simulink model "Vehicle_dynamics"  (R2022a)
settings: Solver=VariableStepAuto  StartTime=0.0  StopTime=20  RelTol=1e-3
undefined symbols (not defined in the file or in its folder): deg, driving, rad, s
libraries: drivingscenarioandsensors x2, simulink_extras x2, autolibshared x2, aerolibconvert2 x1, vehdynlibsteering x1
settings Model: Creator=User  LastModifiedBy=User

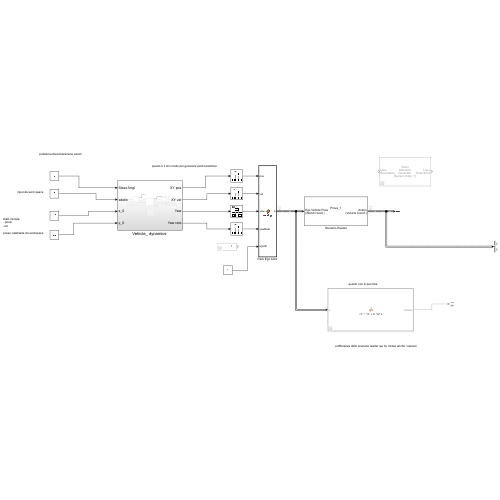
[thumbnail: Simulink's stored preview of the top-level diagram]
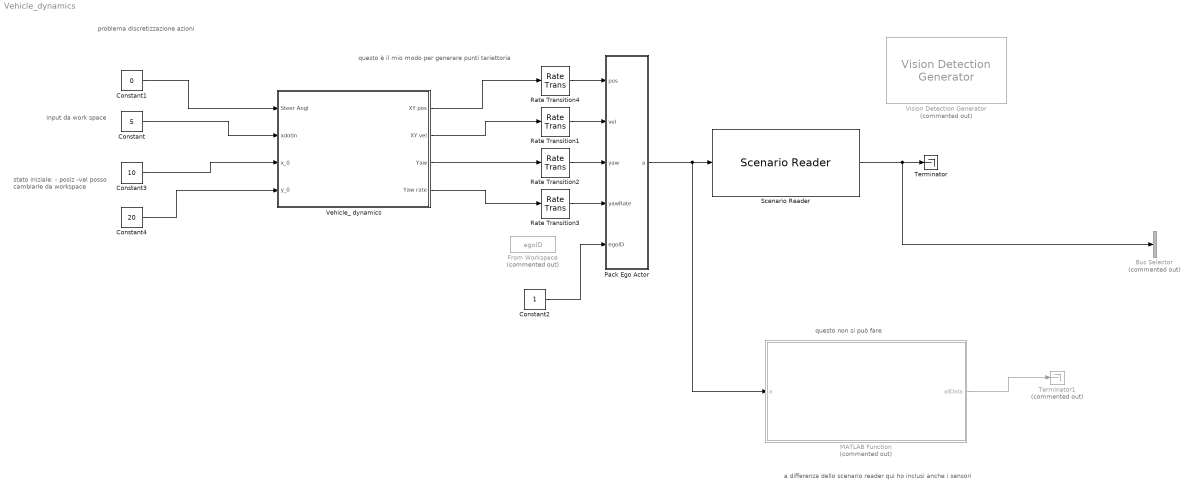
== system Vehicle_dynamics ==
  note: input da work space
  note: questo è il mio modo per generare punti tariettoria
  note: questo non si può fare
  note: a differenza dello scenario reader qui ho inclusi anche i sensori
  note: problema discretizzazione azioni
  note: stato iniziale:
      | - posiz
      | -vel
      |
      | posso cambiarle da workspace
  Bus Selector : BusSelector  Commented=on  OutputSignals=signal1,signal2
  Constant : Constant  Value=5
  Constant1 : Constant  Value=0
  Constant2 : Constant
  Constant3 : Constant  Value=10
  Constant4 : Constant  Value=20
  From Workspace : FromWorkspace  Commented=on  VariableName=egoID
  MATLAB Function : MATLAB Function  Commented=on  TreatAsAtomicUnit=on
  Pack Ego Actor : MATLAB Function  TreatAsAtomicUnit=on
  Rate Transition{1..4} (4 alike) : RateTransition  OutPortSampleTime=Ts
  Scenario Reader : drivingscenarioandsensors/Scenario Reader  ScenarioSource=From file  ScenarioFileName=C:\Users\User\OneDrive\Desktop\Thesis\Codice\Prova_1.mat  ScenarioVariableName=scenario  OutputCoordinateSystem=Vehicle coordinates  EgoVehicleSource=Input port  EgoVehicleActorID=1  OrientVehiclesOnRoad=off  OutputEgoVehiclePose=off  OutputEgoVehicleState=off  SampleTime=0.1  LaneBoundaryOutput=None  LaneBoundaryDistance=0:0.5:9.5  LaneBoundaryLocation=Center of lane markings  BusNameSource=Auto  BusName=BusActors  BusNumActorsSource=Scenario  BusNumActors=100  BusName2Source=Auto  BusName2=BusLaneBoundaries  BusNumLaneBoundariesSource=Scenario  BusNumLaneBoundaries=10  BusName3Source=Auto  BusName3=BusEgoActor  BusName4Source=Auto  BusName4=BusEgoState  ShowCoordinateLabels=on  SimulateUsing=Interpreted execution
  Terminator : Terminator
  Terminator1 : Terminator  Commented=on
  "Vehicle_ dynamics " : Subsystem
  Vision Detection Generator : drivingscenarioandsensors/Vision Detection Generator  Commented=on  SensorIndex=1  DetectorOutput=Lanes only  UpdateInterval=0.1  LaneUpdateInterval=0.1  SensorLocation=[ 1.9, 0 ]  Height=1.1  Yaw=0  Pitch=1  Roll=0  BusNameSource=Auto  BusName=BusObjectDetections  BusName2Source=Auto  BusName2=BusLaneDetections  MaxNumDetectionsSource=Property  MaxNumDetections=50  MaxNumLanesSource=Property  MaxNumLanes=30  DetectionCoordinates=Ego Cartesian  SimulateUsing=Interpreted execution  MaxRange=150  BoundingBoxAccuracy=5  ProcessNoiseIntensity=5  MaxSpeed=100  MaxAllowedOcclusion=0.5  MinObjectImageSize=[ 15, 15 ]  DetectionProbability=0.9  FalsePositivesPerImage=0.1  MinLaneImageSize=[ 20, 3 ]  LaneBoundaryAccuracy=3  HasNoise=on  InitialSeedSource=Repeatable  InitialSeed=0  UsedSeed=driving.internal.SimulinkUtilities.seedManager(gcb)  ActorProfilesSource=From Scenario Reader block  ActorProfilesParameters=driving.internal.ActorProfilesParameters  ActorProfilesExpression=struct( 'ClassID', 0, 'Length', 4.7, 'Width', 1.8, 'Height', 1.4, 'OriginOffset', [ -1.35, 0, 0 ] )  Intrinsics=driving.internal.cameraIntrinsics
  wires:
  Constant1/1 -> "Vehicle_ dynamics "/1(Steer Angl)
  Constant/1 -> "Vehicle_ dynamics "/2(xdotin)
  Rate Transition4/1 -> Pack Ego Actor/1(pos)
  Rate Transition1/1 -> Pack Ego Actor/2(vel)
  Rate Transition2/1 -> Pack Ego Actor/3(yaw)
  Rate Transition3/1 -> Pack Ego Actor/4(yawRate)
  "Vehicle_ dynamics "/1(XY pos) -> Rate Transition4/1
  "Vehicle_ dynamics "/2(XY vel) -> Rate Transition1/1
  "Vehicle_ dynamics "/4(Yaw rate) -> Rate Transition3/1
  Constant2/1 -> Pack Ego Actor/5(egoID)
  "Vehicle_ dynamics "/3(Yaw) -> Rate Transition2/1
  Pack Ego Actor/1(a) -> MATLAB Function/1(a), Scenario Reader/1
  Scenario Reader/1 -> Bus Selector/1, Terminator/1
  Constant3/1 -> "Vehicle_ dynamics "/3(x_0)
  Constant4/1 -> "Vehicle_ dynamics "/4(y_0)
  MATLAB Function/1(allData) -> Terminator1/1

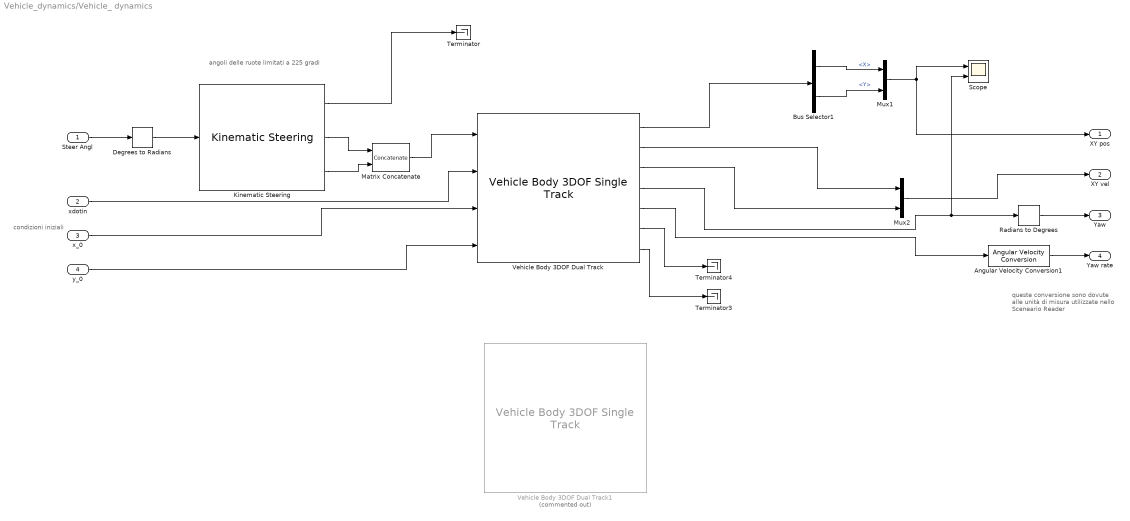
== system Vehicle_dynamics/Vehicle_ dynamics  ==
  note: angoli delle ruote limitati a 225 gradi
  note: condizioni
      | iniziali
  note: queste conversione sono dovute
      | alle unità di misura utilizzate nello
      | Sceneario Reader
  Steer Angl : Inport
  xdotin : Inport  Port=2
  x_0 : Inport  Port=3
  y_0 : Inport  Port=4
  Angular Velocity Conversion1 : aerolibconvert2/Angular Velocity Conversion  IU=rad/s  OU=deg/s
  Bus Selector1 : BusSelector  OutputSignals=InertFrm.Cg.Disp.X,InertFrm.Cg.Disp.Y
  Degrees to Radians : simulink_extras/Transformations/Degrees to Radians
  Kinematic Steering : vehdynlibsteering/Kinematic Steering  StrgType=Ackerman  StrgRatioType=Constant  Loc=Front  NrmlFctr=0.01  TrckWdth=1  WhlBase=1.524  Db=0  StrgRng=1.25*pi  StrgAngBpts="[-6.2832   -5.0265   -3.7699   -2.5133   -1.2566         0    1.2566    2.5133    3.7699    5.0265    6.2832]"  StrgRatioTbl=|  StrgRatio=100  PctAckIn=off  PctAck=100  PctAckTbl=ones(1,11)*100  StrgArmLngth=0.1  RckCsLngth=0.5  TieRodLngth=0.248  D=0.2  PnnRadius=0.00085818  PnnRadiusTbl="[0.0055    0.0055    0.0056    0.0057    0.0058    0.0057    0.0057    0.0057    0.0056    0.0055    0.0055]"  RodLngth=0.1  ParaArmLngth=0.9  aMode=2
      | [13.5000   13.3750   13.2500   13.1250   13.0000   13.0000   13.0000   13.1250   13.2500   13.3750   13.5000
      | ]
  Matrix Concatenate : Concatenate  ConcatenateDimension=2
  Mux1 : Mux  Inputs=2
  Mux2 : Mux  Inputs=2
  Radians to Degrees : simulink_extras/Transformations/Radians to Degrees
  Scope : Scope  NumInputPorts=2
  Terminator : Terminator
  Terminator3 : Terminator
  Terminator4 : Terminator
  Vehicle Body 3DOF Dual Track : autolibshared/Vehicle Body 3DOF Single Track  trackMode=Dual  inputMode=External longitudinal velocity  frontSteerMode=on  rearSteerMode=off  windMode=off  muMode=off  extFMode=off  extMMode=off  htchFMode=off  htchMMode=off  extXo=on  extpsio=off  extxdoto=off  extro=off  extYo=on  extTamb=off  extydoto=off  aMode=2  NF=2  NR=2  m=2000  a=1.4  b=1.6  h=0.35  dh=1  hh=0.2  X_o=0  xdot_o=0  CalphaMode=off  sigmaMode=on  d=0  hl=0  w=[1.4,1.4]  Cy_f=12e3  Cy_r=11e3  sigma_f=.1  sigma_r=.1  alpha_f_brk=[-.1 .1]  Cy_f_data=[-9e3 9e3]  alpha_r_brk=[-.1 .1]  Cy_r_data=[-9e3 9e3]  Y_o=0  ydot_o=0  Izz=4000  psi_o=0  r_o=0  Af=2  Cd=.3  Cl=.1  Cpm=.1  beta_w=[0 0.01:0.01:0.3]  Cs=[0:0.03:0.9]  Cym=[0 1e-6:0.01:0.3]  Pabs=101325  Tair=273  g=9.81  mu=1  xdot_tol=.01  Fznom=5000  Fxtire_sat=7e4  Fytire_sat=7e4  longOff=0  latOff=0  vertOff=0  wrapAng=off
      settings: SourceProductBaseCode=PW,DR,MT,VE
  Vehicle Body 3DOF Dual Track1 : autolibshared/Vehicle Body 3DOF Single Track  Commented=on  trackMode=Dual  inputMode=External longitudinal forces  frontSteerMode=on  rearSteerMode=off  windMode=off  muMode=off  extFMode=off  extMMode=off  htchFMode=off  htchMMode=off  extXo=on  extpsio=off  extxdoto=on  extro=off  extYo=on  extTamb=off  extydoto=off  aMode=2  NF=2  NR=2  m=2000  a=1.4  b=1.6  h=0.35  dh=1  hh=0.2  X_o=0  xdot_o=0  CalphaMode=off  sigmaMode=on  d=0  hl=0  w=[1.4,1.4]  Cy_f=12e3  Cy_r=11e3  sigma_f=.1  sigma_r=.1  alpha_f_brk=[-.1 .1]  Cy_f_data=[-9e3 9e3]  alpha_r_brk=[-.1 .1]  Cy_r_data=[-9e3 9e3]  Y_o=0  ydot_o=0  Izz=4000  psi_o=0  r_o=0  Af=2  Cd=.3  Cl=.1  Cpm=.1  beta_w=[0 0.01:0.01:0.3]  Cs=[0:0.03:0.9]  Cym=[0 1e-6:0.01:0.3]  Pabs=101325  Tair=273  g=9.81  mu=1  xdot_tol=.01  Fznom=5000  Fxtire_sat=7e4  Fytire_sat=7e4  longOff=0  latOff=0  vertOff=0  wrapAng=off
      settings: SourceProductBaseCode=PW,DR,MT,VE
  XY pos : Outport
  XY vel : Outport  Port=2
  Yaw : Outport  Port=3
  Yaw rate : Outport  Port=4
  wires:
  Vehicle Body 3DOF Dual Track/3 -> Mux2/2
  Bus Selector1/2 -> Mux1/2  "<Y>"
  Kinematic Steering/3 -> Matrix Concatenate/2
  Matrix Concatenate/1 -> Vehicle Body 3DOF Dual Track/1
  Vehicle Body 3DOF Dual Track/6 -> Terminator4/1
  Mux1/1 -> XY pos/1, Scope/1
  Vehicle Body 3DOF Dual Track/2 -> Mux2/1
  Vehicle Body 3DOF Dual Track/1 -> Bus Selector1/1
  Bus Selector1/1 -> Mux1/1  "<X>"
  Kinematic Steering/1 -> Terminator/1
  Degrees to Radians/1 -> Kinematic Steering/1
  Vehicle Body 3DOF Dual Track/7 -> Terminator3/1
  Kinematic Steering/2 -> Matrix Concatenate/1
  Mux2/1 -> XY vel/1
  Steer Angl/1 -> Degrees to Radians/1
  xdotin/1 -> Vehicle Body 3DOF Dual Track/2
  Vehicle Body 3DOF Dual Track/4 -> Radians to Degrees/1, Scope/2
  Vehicle Body 3DOF Dual Track/5 -> Angular Velocity Conversion1/1
  Radians to Degrees/1 -> Yaw/1
  Angular Velocity Conversion1/1 -> Yaw rate/1
  x_0/1 -> Vehicle Body 3DOF Dual Track/3
  y_0/1 -> Vehicle Body 3DOF Dual Track/4

== matlab function Vehicle_dynamics/MATLAB Function ==
  data: allData output; a input
function allData  = parking_Scenario(a)
%  function [allData, scenario, sensors] = parking_Scenario(a)

%parking_Scenario - Returns sensor detections
%    allData = parking_Scenario returns sensor detections in a structure
%    with time for an internally defined scenario and sensor suite.
%
%    [allData, scenario, sensors] = parking_Scenario optionally returns
%    the drivingScenario and detection generator objects.

% Generated by MATLAB(R) 9.12 (R2022a) and Automated Driving Toolbox 3.5 (R2022a).
% Generated on: 26-Jul-2022 18:10:48

% Create the drivingScenario object and ego car
[scenario, egoVehicle] = createDrivingScenario;

% Create all the sensors
[sensors, numSensors] = createSensors(scenario);

allData = struct('Time', {}, 'ActorPoses', {}, 'ObjectDetections', {}, 'LaneDetections', {}, 'PointClouds', {}, 'INSMeasurements', {});
% Generate the target poses of all actors relative to the ego vehicle
poses = targetPoses(egoVehicle);
time  = scenario.SimulationTime;

objectDetections = {};
laneDetections   = [];
ptClouds = {};
insMeas = {};
isValidTime = false(1, numSensors);
isValidLaneTime = false(1, numSensors);
isValidPointCloudTime = false(1, numSensors);
isValidINSTime = false(1, numSensors);

% Generate detections for each sensor
for sensorIndex = 1:numSensors
    sensor = sensors{sensorIndex};
    % Generate the ego vehicle lane boundaries
    if isa(sensor, 'visionDetectionGenerator')
        maxLaneDetectionRange = min(500,sensor.MaxRange);
        lanes = laneBoundaries(egoVehicle, 'XDistance', linspace(-maxLaneDetectionRange, maxLaneDetectionRange, 101));
    end
    type = getDetectorOutput(sensor);
    if strcmp(type, 'Objects only')
        if isa(sensor,'ultrasonicDetectionGenerator')
            [objectDets, isValidTime(sensorIndex)] = sensor(poses, time);
            numObjects = length(objectDets);
        else
            [objectDets, numObjects, isValidTime(sensorIndex)] = sensor(poses, time);
        end
        objectDetections = [objectDetections; objectDets(1:numObjects)];
    elseif strcmp(type, 'Lanes only')
        [laneDets, ~, isValidTime(sensorIndex)] = sensor(lanes, time);
        laneDetections   = [laneDetections laneDets];
    elseif strcmp(type, 'Lanes and objects')
        [objectDets, numObjects, isValidTime(sensorIndex), laneDets, ~, isValidLaneTime(sensorIndex)] = sensor(poses, lanes, time);
        objectDetections = [objectDetections; objectDets(1:numObjects)];
        laneDetections   = [laneDetections laneDets];
    elseif strcmp(type, 'Lanes with occlusion')
        [laneDets, ~, isValidLaneTime(sensorIndex)] = sensor(poses, lanes, time);
        laneDetections   = [laneDetections laneDets];
    elseif strcmp(type, 'PointCloud')
        if sensor.HasRoadsInputPort
            rdmesh = roadMesh(egoVehicle,min(500,sensor.MaxRange));
            [ptCloud, isValidPointCloudTime(sensorIndex)] = sensor(poses, rdmesh, time);
        else
            [ptCloud, isValidPointCloudTime(sensorIndex)] = sensor(poses, time);
        end
        ptClouds = [ptClouds; ptCloud];
    elseif strcmp(type, 'INSMeasurement')
        insMeasCurrent = sensor(actorState, time);
        insMeas = [insMeas; insMeasCurrent];
        isValidINSTime(sensorIndex) = true;
    end
end

% Aggregate all detections into a structure for later use
if any(isValidTime) || any(isValidLaneTime) || any(isValidPointCloudTime) || any(isValidINSTime)
    allData(end + 1) = struct( ...
        'Time',       scenario.SimulationTime, ...
        'ActorPoses', actorPoses(scenario), ...
        'ObjectDetections', {objectDetections}, ...
        'LaneDetections', {laneDetections}, ...
        'PointClouds',   {ptClouds}, ...
        'INSMeasurements',   {insMeas});
end

% Release all the sensor objects so they can be used again.
for sensorIndex = 1:numSensors
    release(sensors{sensorIndex});
end

%%%%%%%%%%%%%%%%%%%%
% Helper functions %
%%%%%%%%%%%%%%%%%%%%

% Units used in createSensors and createDrivingScenario
% Distance/Position - meters
% Speed             - meters/second
% Angles            - degrees
% RCS Pattern       - dBsm

function [sensors, numSensors] = createSensors(scenario)
% createSensors Returns all sensor objects to generate detections

% Assign into each sensor the physical and radar profiles for all actors
profiles = actorProfiles(scenario);
sensors{1} = ultrasonicDetectionGenerator('SensorIndex', 1, ...
    'MountingLocation', [2.47 0.01 0.2], ...
    'FieldOfView', [80 35], ...
    'Profiles', profiles);
sensors{2} = ultrasonicDetectionGenerator('SensorIndex', 2, ...
    'MountingLocation', [0.16 -0.02 0.2], ...
    'MountingAngles', [-180 0 0], ...
    'FieldOfView', [80 35], ...
    'Profiles', profiles);
sensors{3} = visionDetectionGenerator('SensorIndex', 3, ...
    'SensorLocation', [1.33 0.9], ...
    'Yaw', 90, ...
    'DetectorOutput', 'Lanes with occlusion', ...
    'Intrinsics', cameraIntrinsics([300 800],[320 240],[480 640]), ...
    'ActorProfiles', profiles);
numSensors = 3;

function [scenario, egoVehicle] = createDrivingScenario
% createDrivingScenario Returns the drivingScenario defined in the Designer

% Construct a drivingScenario object.
scenario = drivingScenario;

% Add all road segments
roadCenters = [0 0 0;
    25 0 0];
marking = [laneMarking('Solid', 'Color', [0.98 0.86 0.36])
    laneMarking('Dashed')];
laneSpecification = lanespec(1, 'Width', 20, 'Marking', marking);
road(scenario, roadCenters, 'Lanes', laneSpecification, 'Name', 'Road');

% Add the actors
vehicle(scenario, ...
    'ClassID', 1, ...
    'Position', [2.05 8.32 0.01], ...
    'Mesh', driving.scenario.carMesh, ...
    'Name', 'Car');

vehicle(scenario, ...
    'ClassID', 1, ...
    'Position', [20.05 8.12 0.01], ...
    'Mesh', driving.scenario.carMesh, ...
    'Name', 'Car1');

% Add the ego vehicle
egoVehicle = vehicle(scenario, ...
    'ClassID', 1, ...
    'Position', [11.4218662404233 3.09486084808245 0.01], ...
    'Mesh', driving.scenario.carMesh, ...
    'Name', 'Car2');

function output = getDetectorOutput(sensor)

if isa(sensor, 'visionDetectionGenerator')
    output = sensor.DetectorOutput;
elseif isa(sensor, 'lidarPointCloudGenerator')
    output = 'PointCloud';
elseif isa(sensor, 'insSensor')
    output = 'INSMeasurement';
else
    output = 'Objects only';
end

== matlab function Vehicle_dynamics/Pack Ego Actor ==
  data: pos input; a output Bus: BusActors1Actors size=1; vel input; yaw input; yawRate input; egoID input
function a = packEgo(pos,vel,yaw,yawRate,egoID)
% Pack ego information into a single ego actor bus
%
% Imoprtant note:
% Output is a bus of type BusActorsActors. This is the same bus used by the
% Scenario Reader to output an individual actor. If you change the
% output bus name of Scenario Reader change the output bus name here
% as well by clicking on 'Edit Data' in the menu above.

a = struct(...
    'ActorID',egoID,...
    'Position', [pos(1) pos(2) 0], ...
    'Velocity', [vel(1) vel(2) 0], ...
    'Roll', 0, ...
    'Pitch', 0, ...
    'Yaw', yaw, ...
    'AngularVelocity', [0 0 yawRate]);
